simulink model "sampleModel1522"  (R2023a)
settings: Solver=VariableStepAuto  StartTime=0.0  StopTime=10.0  RelTol=1e-3
libraries: hdlsllib x4, simulink x1
settings Model: Creator=user1  LastModifiedBy=user1

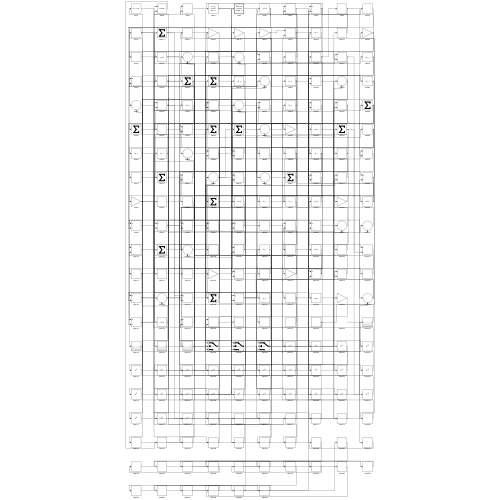
[thumbnail: Simulink's stored preview of the top-level diagram]
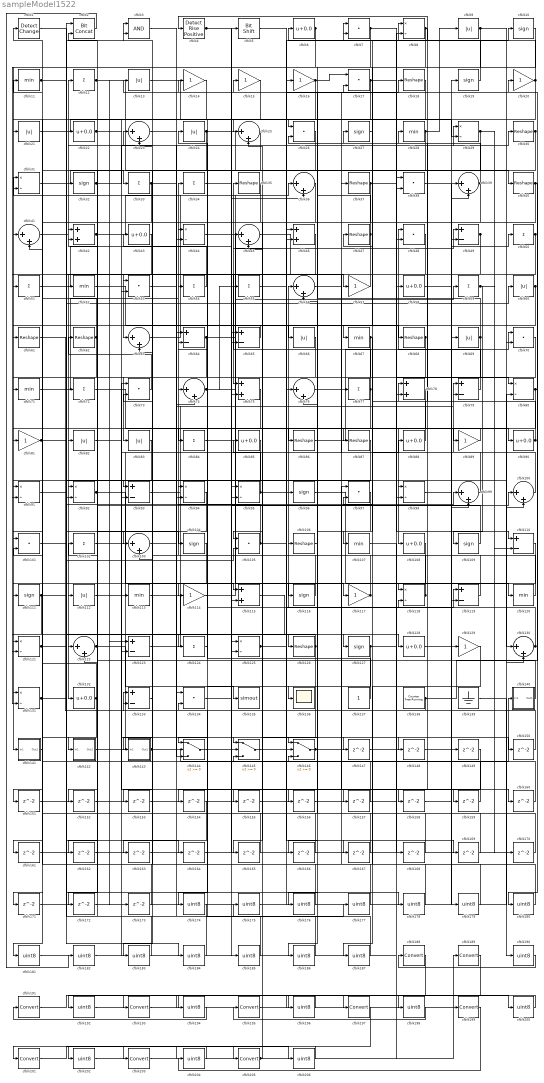
== system sampleModel1522 ==
  cfblk1 : simulink/Logic and Bit Operations/Detect Change  vinit=0  OutDataTypeStr=boolean
      settings: LibrarySourceBlock=|
      | hdlsllib/Logic and Bit
      | Operations/Detect
      | Change
  cfblk{10,19,27,32,96,104,109,111,116,127} (10 alike) : Signum
  cfblk{23,25,36,39,41,45,56,63,74,76,99..100,103,122,130} (15 alike) : Sum  Inputs=|++
  cfblk{7,17,26,38,48,53,70,73,97,101,105,134} (12 alike) : DotProduct  OutDataTypeStr=Inherit: Inherit via internal rule
  cfblk{12,33..34,50..51,54..55,59,72,77,84,102,124} (13 alike) : Sum  Inputs=+
  cfblk{18,30,35,37,40,47,61..62,68,86..87,106,126} (13 alike) : Reshape
  cfblk{11,28,52,67,71,107,113,120} (8 alike) : MinMax
  cfblk{6,22,43,58,85,88,90,108,128,132} (10 alike) : Bias  Bias=0.0  SaturateOnIntegerOverflow=off
  cfblk{49,64..65,79,93,110,119,123,133} (9 alike) : Sum  Inputs=+-
  cfblk{9,13,21,24,60,66,69,82..83,112} (10 alike) : Abs  SaturateOnIntegerOverflow=off
  cfblk{14..16,20,57,81,89,114,117,129} (10 alike) : Gain
  cfblk{42,46,75,78,115} (5 alike) : Sum
  cfblk{8,29,31,44,80,91..92,94..95,98,118,121,125,131} (14 alike) : Product  Inputs=*/  RndMeth=Zero  SaturateOnIntegerOverflow=on
  cfblk135 : ToWorkspace  VariableName=simout  SaveFormat=Timeseries  SampleTime=-1
  cfblk136 : Scope
  cfblk137 : Constant  SampleTime=-1
  cfblk138 : hdlsllib/Sources/Counter Free-Running  NumBits=16  tsamp=-1
  cfblk139 : Ground
  cfblk140 : Subsystem
      settings: LibrarySourceBlock=|
      | hdlsllib/Ports &
      | Subsystems/Subsystem
  cfblk141 : Subsystem
      settings: LibrarySourceBlock=|
      | hdlsllib/Ports &
      | Subsystems/Subsystem
  cfblk142 : Subsystem
      settings: LibrarySourceBlock=|
      | hdlsllib/Ports &
      | Subsystems/Subsystem
  cfblk143 : Subsystem
      settings: LibrarySourceBlock=|
      | hdlsllib/Ports &
      | Subsystems/Subsystem
  cfblk144 : Switch  SaturateOnIntegerOverflow=off  InputSameDT=off
  cfblk145 : Switch  SaturateOnIntegerOverflow=off  InputSameDT=off
  cfblk146 : Switch  SaturateOnIntegerOverflow=off  InputSameDT=off
  cfblk{147..173} (27 alike) : Delay  SampleTime=1
  cfblk{174..187,190,192,194,196,198,200,202,204,206} (23 alike) : DataTypeConversion  OutDataTypeStr=uint8  SaturateOnIntegerOverflow=off  RndMeth=Floor
  cfblk{188..189,191,193,195,197,199,201,203,205} (10 alike) : DataTypeConversion  SaturateOnIntegerOverflow=off  RndMeth=Floor
  cfblk2 : hdlsllib/Logic and Bit Operations/Bit Concat  numInputs=2
  cfblk3 : Logic  AllPortsSameDT=off  OutDataTypeStr=boolean
  cfblk4 : hdlsllib/Logic and Bit Operations/Detect Rise Positive  vinit=0  OutDataTypeStr=boolean
  cfblk5 : hdlsllib/Logic and Bit Operations/Bit Shift  mode=Shift Left Logical  N=0
  wires:
  cfblk64/1 -> cfblk59/1, cfblk123/2
  cfblk96/1 -> cfblk120/1
  cfblk57/1 -> cfblk132/1
  cfblk130/1 -> cfblk56/1, cfblk94/1
  cfblk62/1 -> cfblk82/1, cfblk11/1
  cfblk138/1 -> cfblk15/1, cfblk133/2
  cfblk22/1 -> cfblk25/1, cfblk147/1
  cfblk119/1 -> cfblk34/1
  cfblk74/1 -> cfblk117/1, cfblk55/1
  cfblk31/1 -> cfblk33/1
  cfblk70/1 -> cfblk83/1
  cfblk77/1 -> cfblk35/1, cfblk155/1
  cfblk142/1(Out1) -> cfblk74/1
  cfblk6/1 -> cfblk141/1(In1), cfblk65/2
  cfblk8/1 -> cfblk41/1, cfblk118/1
  cfblk124/1 -> cfblk24/1
  cfblk41/1 -> cfblk12/1
  cfblk100/1 -> cfblk79/1
  cfblk83/1 -> cfblk92/1
  cfblk122/1 -> cfblk5/1, cfblk135/1
  cfblk117/1 -> cfblk106/1, cfblk31/1
  cfblk43/1 -> cfblk63/1
  cfblk33/1 -> cfblk125/2, cfblk151/1
  cfblk114/1 -> cfblk49/1
  cfblk65/1 -> cfblk61/1
  cfblk88/1 -> cfblk78/1
  cfblk93/1 -> cfblk19/1
  cfblk40/1 -> cfblk119/2, cfblk180/1
  cfblk58/1 -> cfblk69/1
  cfblk16/1 -> cfblk17/1, cfblk144/3
  cfblk20/1 -> cfblk4/1, cfblk78/2, cfblk48/2
  cfblk27/1 -> cfblk7/1
  cfblk61/1 -> cfblk133/1
  cfblk146/1 -> cfblk39/2, cfblk98/2
  cfblk32/1 -> cfblk30/1, cfblk160/1
  cfblk29/1 -> cfblk112/1, cfblk110/2
  cfblk72/1 -> cfblk108/1
  cfblk42/1 -> cfblk36/1, cfblk123/1
  cfblk115/1 -> cfblk128/1
  cfblk12/1 -> cfblk130/1, cfblk173/1
  cfblk44/1 -> cfblk86/1
  cfblk85/1 -> cfblk131/1
  cfblk79/1 -> cfblk48/1
  cfblk89/1 -> cfblk81/1
  cfblk84/1 -> cfblk16/1
  cfblk95/1 -> cfblk85/1, cfblk167/1
  cfblk54/1 -> cfblk23/1
  cfblk55/1 -> cfblk17/2
  cfblk52/1 -> cfblk68/1
  cfblk123/1 -> cfblk46/1
  cfblk49/1 -> cfblk146/1, cfblk53/2
  cfblk39/1 -> cfblk71/1, cfblk51/1, cfblk26/2
  cfblk25/1 -> cfblk53/1
  cfblk81/1 -> cfblk104/1, cfblk184/1
  cfblk140/1(Out1) -> cfblk102/1
  cfblk35/1 -> cfblk92/2
  cfblk36/1 -> cfblk105/1
  cfblk63/1 -> cfblk8/1
  cfblk86/1 -> cfblk70/1
  cfblk113/1 -> cfblk127/1
  cfblk68/1 -> cfblk122/1, cfblk93/2
  cfblk11/1 -> cfblk57/1, cfblk100/2
  cfblk28/1 -> cfblk143/1(In1), cfblk9/1
  cfblk7/1 -> cfblk80/1, cfblk156/1
  cfblk71/1 -> cfblk54/1
  cfblk59/1 -> cfblk109/1, cfblk170/1
  cfblk126/1 -> cfblk121/1, cfblk165/1
  cfblk50/1 -> cfblk124/1, cfblk91/2, cfblk52/1
  cfblk3/1 -> cfblk145/1
  cfblk21/1 -> cfblk26/1
  cfblk73/1 -> cfblk62/1
  cfblk128/1 -> cfblk129/1
  cfblk91/1 -> cfblk126/1
  cfblk24/1 -> cfblk96/1, cfblk101/1
  cfblk144/1 -> cfblk100/1
  cfblk102/1 -> cfblk37/1
  cfblk19/1 -> cfblk6/1
  cfblk92/1 -> cfblk115/1, cfblk150/1
  cfblk103/1 -> cfblk79/2
  cfblk48/1 -> cfblk116/1
  cfblk111/1 -> cfblk99/1, cfblk131/2
  cfblk109/1 -> cfblk42/1
  cfblk56/1 -> cfblk18/1
  cfblk127/1 -> cfblk10/1, cfblk154/1
  cfblk78/1 -> cfblk103/1
  cfblk60/1 -> cfblk144/1, cfblk84/1, cfblk166/1
  cfblk112/1 -> cfblk88/1
  cfblk75/1 -> cfblk142/1(In1)
  cfblk45/1 -> cfblk77/1
  cfblk118/1 -> cfblk45/1, cfblk111/1
  cfblk67/1 -> cfblk87/1, cfblk115/2
  cfblk46/1 -> cfblk75/1
  cfblk82/1 -> cfblk98/1
  cfblk120/1 -> cfblk22/1
  cfblk125/1 -> cfblk119/1, cfblk118/2, cfblk169/1
  cfblk10/1 -> cfblk67/1
  cfblk30/1 -> cfblk76/2, cfblk158/1
  cfblk53/1 -> cfblk64/1
  cfblk80/1 -> cfblk95/2, cfblk20/1, cfblk107/1
  cfblk17/1 -> cfblk90/1, cfblk44/2
  cfblk13/1 -> cfblk65/1
  cfblk99/1 -> cfblk27/1
  cfblk51/1 -> cfblk36/2
  cfblk47/1 -> cfblk66/1, cfblk14/1
  cfblk18/1 -> cfblk114/1
  cfblk98/1 -> cfblk50/1
  cfblk9/1 -> cfblk70/2, cfblk121/2
  cfblk34/1 -> cfblk89/1
  cfblk131/1 -> cfblk3/1, cfblk60/1
  cfblk143/1(Out1) -> cfblk140/1(In1), cfblk103/2, cfblk29/1, cfblk163/1
  cfblk69/1 -> cfblk13/1, cfblk94/2
  cfblk116/1 -> cfblk32/1
  cfblk106/1 -> cfblk136/1
  cfblk137/1 -> cfblk64/2
  cfblk132/1 -> cfblk101/2, cfblk171/1
  cfblk26/1 -> cfblk122/2
  cfblk5/1 -> cfblk76/1
  cfblk4/1 -> cfblk145/2, cfblk29/2
  cfblk133/1 -> cfblk3/2
  cfblk14/1 -> cfblk21/1
  cfblk37/1 -> cfblk93/1, cfblk110/1
  cfblk105/1 -> cfblk44/1, cfblk148/1
  cfblk23/1 -> cfblk40/1
  cfblk101/1 -> cfblk72/1
  cfblk66/1 -> cfblk91/1
  cfblk90/1 -> cfblk28/1, cfblk47/1
  cfblk121/1 -> cfblk105/2, cfblk164/1
  cfblk147/1 -> cfblk39/1
  cfblk148/1 -> cfblk49/2
  cfblk150/1 -> cfblk73/2
  cfblk151/1 -> cfblk74/2
  cfblk104/1 -> cfblk152/1
  cfblk152/1 -> cfblk46/2
  cfblk87/1 -> cfblk153/1
  cfblk153/1 -> cfblk8/2
  cfblk155/1 -> cfblk45/2
  cfblk156/1 -> cfblk56/2
  cfblk145/1 -> cfblk157/1
  cfblk157/1 -> cfblk63/2
  cfblk158/1 -> cfblk99/2
  cfblk76/1 -> cfblk159/1
  cfblk159/1 -> cfblk41/2
  cfblk160/1 -> cfblk144/2
  cfblk141/1(Out1) -> cfblk161/1
  cfblk161/1 -> cfblk95/1
  cfblk110/1 -> cfblk162/1
  cfblk162/1 -> cfblk75/2
  cfblk163/1 -> cfblk80/2
  cfblk164/1 -> cfblk125/1
  cfblk165/1 -> cfblk42/2
  cfblk166/1 -> cfblk31/2
  cfblk167/1 -> cfblk25/2
  cfblk107/1 -> cfblk168/1
  cfblk168/1 -> cfblk7/2
  cfblk169/1 -> cfblk146/3
  cfblk170/1 -> cfblk23/2
  cfblk171/1 -> cfblk146/2
  cfblk94/1 -> cfblk172/1
  cfblk172/1 -> cfblk130/2
  cfblk173/1 -> cfblk1/1
  cfblk149/1 -> cfblk174/1
  cfblk175/1 -> cfblk149/1
  cfblk97/1 -> cfblk176/1
  cfblk176/1 -> cfblk43/1
  cfblk174/1 -> cfblk177/1
  cfblk177/1 -> cfblk97/1
  cfblk1/1 -> cfblk178/1
  cfblk178/1 -> cfblk97/2
  cfblk38/1 -> cfblk179/1
  cfblk179/1 -> cfblk73/1
  cfblk180/1 -> cfblk38/1
  cfblk15/1 -> cfblk181/1
  cfblk181/1 -> cfblk38/2
  cfblk2/1 -> cfblk182/1
  cfblk182/1 -> cfblk113/1
  cfblk154/1 -> cfblk183/1
  cfblk183/1 -> cfblk2/1
  cfblk184/1 -> cfblk2/2
  cfblk134/1 -> cfblk185/1
  cfblk185/1 -> cfblk175/1
  cfblk108/1 -> cfblk186/1
  cfblk186/1 -> cfblk134/1
  cfblk129/1 -> cfblk187/1
  cfblk187/1 -> cfblk134/2
  cfblk139/1 -> cfblk190/1
  cfblk190/1 -> cfblk188/1
  cfblk188/1 -> cfblk192/1
  cfblk192/1 -> cfblk189/1
  cfblk189/1 -> cfblk194/1
  cfblk194/1 -> cfblk191/1
  cfblk191/1 -> cfblk196/1
  cfblk196/1 -> cfblk193/1
  cfblk193/1 -> cfblk198/1
  cfblk198/1 -> cfblk195/1
  cfblk195/1 -> cfblk200/1
  cfblk200/1 -> cfblk197/1
  cfblk197/1 -> cfblk202/1
  cfblk202/1 -> cfblk199/1
  cfblk203/1 -> cfblk205/1
  cfblk199/1 -> cfblk204/1
  cfblk204/1 -> cfblk201/1
  cfblk205/1 -> cfblk145/3, cfblk58/1
  cfblk201/1 -> cfblk206/1
  cfblk206/1 -> cfblk203/1

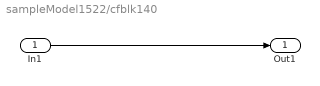
== system sampleModel1522/cfblk140 ==
  In1 : Inport
  Out1 : Outport
  wires:
  In1/1 -> Out1/1

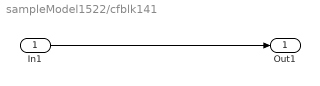
== system sampleModel1522/cfblk141 ==
  In1 : Inport
  Out1 : Outport
  wires:
  In1/1 -> Out1/1

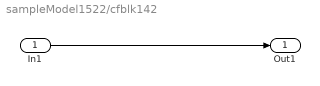
== system sampleModel1522/cfblk142 ==
  In1 : Inport
  Out1 : Outport
  wires:
  In1/1 -> Out1/1

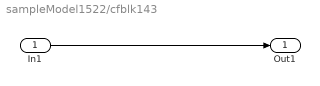
== system sampleModel1522/cfblk143 ==
  In1 : Inport
  Out1 : Outport
  wires:
  In1/1 -> Out1/1
